simulink model "sampleModel349"  (R2021b)
settings: Solver=VariableStepAuto  StartTime=0.0  StopTime=10.0  RelTol=1e-3
undefined symbols (not defined in the file or in its folder): Newton, Raphson
libraries: simulink x12, slpidlib x2, simulink_need_slupdate x2
settings Model: Creator=user  LastModifiedBy=user

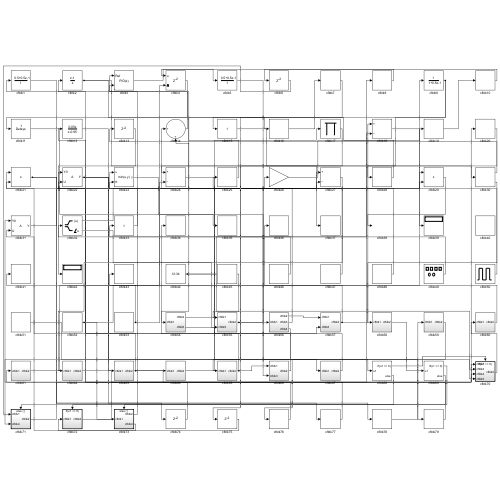
[thumbnail: Simulink's stored preview of the top-level diagram]
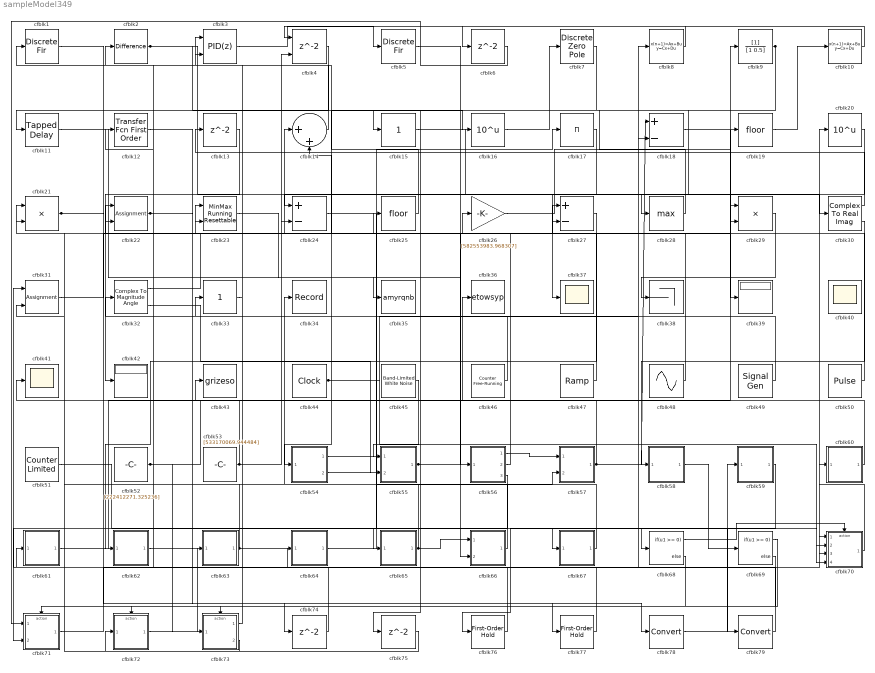
== system sampleModel349 ==
  cfblk1 : DiscreteFir  SampleTime=1
  cfblk10 : DiscreteStateSpace
  cfblk11 : simulink/Discrete/Tapped Delay  vinit=0.0  samptime=-1  NumDelays=1  DelayOrder=Oldest  includeCurrent=off
  cfblk12 : simulink/Discrete/Transfer Fcn First Order  PoleZ=0.95  ICPrevOutput=0.0  DoSatur=off
  cfblk{6,13,74..75} (4 alike) : Delay  SampleTime=1
  cfblk14 : Sum  Inputs=|++
  cfblk15 : simulink/Math Operations/Slider Gain  gain=1  low=0  high=2
  cfblk16 : Math  Operator=10^u  SaturateOnIntegerOverflow=on
  cfblk17 : Product  Inputs=*
  cfblk18 : Sum  Inputs=+-
  cfblk19 : Rounding
  cfblk2 : simulink/Discrete/Difference  ICPrevInput=0.0  OutMin=[]  OutMax=[]  OutDataTypeStr=Inherit: Inherit via back propagation  OutDataType=fixdt(1, 16)  OutScaling=2^-10  DoSatur=off
  cfblk20 : Math  Operator=10^u  SaturateOnIntegerOverflow=on
  cfblk21 : Product
  cfblk22 : Assignment  DiagnosticForDimensions=Warning  IndexOptions=Index vector (dialog)  Indices=1  OutputSizes=1
  cfblk23 : simulink/Math Operations/MinMax Running Resettable  Function=min  vinit=0.0
  cfblk24 : Sum  Inputs=+-
  cfblk25 : Rounding
  cfblk26 : Gain  Gain=[582553983.968307]
  cfblk27 : Sum  Inputs=+-
  cfblk28 : MinMax  Function=max
  cfblk29 : Product
  cfblk3 : slpidlib/PID Controller (2DOF)  Controller=PID  Form=Parallel  TimeDomain=Discrete-time  UseExternalTs=off  SampleTime=1  IntegratorMethod=Forward Euler  FilterMethod=Forward Euler  ControllerParametersSource=internal  P=1  I=1  D=0  UseFilter=on  N=100  b=1  c=1  TunerSelectOption=Transfer Function Based (PID Tuner App)  InitialConditionSource=internal  InitialConditionForIntegrator=0  InitialConditionForFilter=0  DifferentiatorICPrevScaledInput=0  ExternalReset=none  TrackingMode=off  Kt=1  LimitOutput=off  SatLimitsSource=internal  UpperSaturationLimit=inf  LowerSaturationLimit=-inf  LinearizeAsGain=off  AntiWindupMode=none  Kb=1  POutMin=[]  POutMax=[]  IOutMin=[]  IOutMax=[]  DOutMin=[]  DOutMax=[]  NOutMin=[]  NOutMax=[]  bOutMin=[]  bOutMax=[]  cOutMin=[]  cOutMax=[]  SumOutMin=[]  SumOutMax=[]  SaturationOutMin=[]  SaturationOutMax=[]  PParamMin=[]  PParamMax=[]  IParamMin=[]  IParamMax=[]  DParamMin=[]  DParamMax=[]  NParamMin=[]  NParamMax=[]  bParamMin=[]  bParamMax=[]  cParamMin=[]  cParamMax=[]  KbParamMin=[]  KbParamMax=[]  KtParamMin=[]  KtParamMax=[]  KbOutMin=[]  KbOutMax=[]  KtOutMin=[]  KtOutMax=[]  IntegratorOutMin=[]  IntegratorOutMax=[]  FilterOutMin=[]  FilterOutMax=[]  SumI1OutMin=[]  SumI1OutMax=[]  SumI2OutMin=[]  SumI2OutMax=[]  SumI3OutMin=[]  SumI3OutMax=[]  SumI4OutMin=[]  SumI4OutMax=[]  SumDOutMin=[]  SumDOutMax=[]  Sum1OutMin=[]  Sum1OutMax=[]  Sum2OutMin=[]  Sum2OutMax=[]  Sum3OutMin=[]  Sum3OutMax=[]  DifferentiatorOutMin=[]  DifferentiatorOutMax=[]  FilterDiffOutCoefMin=[]  FilterDiffOutCoefMax=[]  ReciprocalOutMin=[]  ReciprocalOutMax=[]  SumDenOutMin=[]  SumDenOutMax=[]  SumNumOutMin=[]  SumNumOutMax=[]  DivideOutMin=[]  DivideOutMax=[]  UdiffTsProdOutMin=[]  UdiffTsProdOutMax=[]  NTsProdOutMin=[]  NTsProdOutMax=[]  UintegralTsProdOutMin=[]  UintegralTsProdOutMax=[]  UngainTsProdOutMin=[]  UngainTsProdOutMax=[]  IntegratorContinuousStateAttributes=''  IntegratorStateMustResolveToSignalObject=off  IntegratorRTWStateStorageClass=Auto  FilterContinuousStateAttributes=''  FilterStateMustResolveToSignalObject=off  FilterRTWStateStorageClass=Auto  ParallelPVariant=InternalParameters  IdealPVariant=Disabled  IVariant=InternalParameters  DVariant=InternalParameters  bVariant=InternalParameters  cVariant=InternalParameters  IntegratorVariant=Discrete  SatVariant=Disabled  AWVariant=Passthrough  PCopyVariant=Disabled  TRVariant=Disabled  FdbkBlocksVariant=Forward  IdealPFdbkVariant=Disabled  SatFdbkVariant=Disabled  DerivativeFilterVariant=ForwardEulerFilter  NVariant=InternalParameters  NCopyVariant=Disabled  FilterICVariant=InternalICsFilter  IntegratorICVariant=InternalICs  ExternalResetVariant=Disabled  TRSumVariant=Passthrough  SumFdbkVariant=Disabled  SumVariant=Sum_PID  TsampFilterVariant=InternalTs  TsampNgainVariant=Passthrough  TsampIntegralVariant=Passthrough  ExternalSaturationOutDataTypeStr=Inherit: Same as second input
      settings: SourceProductBaseCode=SL
  cfblk30 : ComplexToRealImag
  cfblk31 : Assignment  DiagnosticForDimensions=Warning  IndexOptions=Index vector (dialog)  Indices=1  OutputSizes=1
  cfblk32 : ComplexToMagnitudeAngle
  cfblk33 : simulink/Math Operations/Slider Gain  gain=1  low=0  high=2
  cfblk34 : Record  FileSettingsInternal="{\"entries\":[{\"content\":{\"excelSettings\":{\"content\":{},\"type\":\"Streamout.ExcelSettings\"}},\"type\":\"Streamout.FileSettingStorage\",\"uuid\":\"f71aceab-5a60-49d6-a025-645f4f33ca44\"}],\"packageUris\":[\"http://schema.mathworks.com/mf0/streamout_blocks/R2020a\"],\"version\":\"1.0\"}"  SignalsInternal="{\"entries\":[{\"content\":{\"signals\":[{\"content\":{\"blockPath\":[\"sampleModel349/cfblk34\"],\"channel\":[],\"dimensions\":[1],\"domain\":\"sampleModel349/cfblk34\",\"lineColor\":\"#d95319\",\"plots\":[1],\"port\":1,\"sid\":[\"\"],\"signalID\":14601,\"signalName\":\"cfblk67\"},\"type\":\"RecordBlkView.Signal\",\"uuid\":\"4f28f7ec-e5ea-41ac-ba8a-1c5bf7ad2562\"}]},\"type\":\"RecordBlkView.InputSignals\",\"uuid\":\"3db0044d-db04-4044-a744-d9451d8b6dbf\"}],\"packageUris\":[\"http://schema.mathworks.com/mf0/streamout_blocks/R2020a\"],\"version\":\"1.0\"}"  VisualizationBindings="{\"sparklinesplugin\":{\"info\":[{\"bindingParametersList\":[],\"subplotID\":1}]}}"
  cfblk35 : ToWorkspace  VariableName=amyrqnb  SaveFormat=Timeseries  SampleTime=-1
  cfblk36 : ToWorkspace  VariableName=etowsyp  SaveFormat=Timeseries  SampleTime=-1
  cfblk37 : Scope
  cfblk38 : Terminator
  cfblk39 : Display
  cfblk4 : Delay  ShowEnablePort=on  SampleTime=1
      settings: InputPortMap=u0,e6
  cfblk40 : Scope
      settings: Floating=on
  cfblk41 : Scope
  cfblk42 : Display
  cfblk43 : ToWorkspace  VariableName=grizeso  SaveFormat=Timeseries  SampleTime=-1
  cfblk44 : DigitalClock
  cfblk45 : simulink/Sources/Band-Limited White Noise  Cov=[8754681935.924770]  Ts=0.1  seed=[7344934764.000000]
  cfblk46 : simulink/Sources/Counter Free-Running  NumBits=[11.000000]  tsamp=-1
  cfblk47 : simulink/Sources/Ramp  slope=[7962.295624]  start=[45.118669]  InitialOutput=[46132.244628]
  cfblk48 : Sin  Amplitude=[-585222827.413026]  Bias=[408906363.797786]  SampleTime=0
  cfblk49 : SignalGenerator  Amplitude=[-354647075.884674]
  cfblk5 : DiscreteFir  SampleTime=1
  cfblk50 : DiscretePulseGenerator  PulseType=Time based  Amplitude=[-738225747.872744]  Period=[73691068.508407]  PulseWidth=5  PhaseDelay=[9.000000]
  cfblk51 : simulink/Sources/Counter Limited  uplimit=[482.000000]  tsamp=-1
  cfblk52 : Constant  Value=[222412271.325236]  SampleTime=1
  cfblk53 : Constant  Value=[533170069.944484]  SampleTime=1
  cfblk54 : Subsystem
  cfblk55 : Subsystem
  cfblk56 : Subsystem
  cfblk57 : Subsystem
  cfblk58 : Subsystem
  cfblk59 : Subsystem
  cfblk60 : Subsystem
  cfblk61 : Subsystem
  cfblk62 : Subsystem
  cfblk63 : Subsystem
  cfblk64 : Subsystem
  cfblk65 : Subsystem
  cfblk66 : Subsystem
  cfblk67 : Subsystem
  cfblk68 : If  IfExpression=u1 >= 0  SampleTime=1
  cfblk69 : If  IfExpression=u1 >= 0  SampleTime=1
  cfblk7 : DiscreteZeroPole  Poles=[0 0.5]  Gain=1
  cfblk70 : Subsystem  TreatAsAtomicUnit=on
  cfblk71 : Subsystem  TreatAsAtomicUnit=on
  cfblk72 : Subsystem  TreatAsAtomicUnit=on
  cfblk73 : Subsystem  TreatAsAtomicUnit=on
  cfblk76 : simulink_need_slupdate/First-Order Hold  DisableCoverage=on  Ts=1
      settings: SourceProductBaseCode=SL
  cfblk77 : simulink_need_slupdate/First-Order Hold  DisableCoverage=on  Ts=1
      settings: SourceProductBaseCode=SL
  cfblk78 : DataTypeConversion
  cfblk79 : DataTypeConversion
  cfblk8 : DiscreteStateSpace
  cfblk9 : DiscreteFilter  SampleTime=1
  wires:
  cfblk25/1 -> cfblk3/1
  cfblk24/1 -> cfblk68/1
  cfblk46/1 -> cfblk33/1
  cfblk64/1(cfblk2) -> cfblk17/1
  cfblk62/1(cfblk2) -> cfblk20/1
  cfblk55/1(cfblk2) -> cfblk56/1(cfblk1), cfblk27/1
  cfblk10/1 -> cfblk6/1
  cfblk3/1 -> cfblk5/1
  cfblk28/1 -> cfblk15/1
  cfblk13/1 -> cfblk42/1
  cfblk6/1 -> cfblk71/1(cfblk1)
  cfblk5/1 -> cfblk67/1(cfblk1)
  cfblk47/1 -> cfblk14/1
  cfblk54/1(cfblk2) -> cfblk26/1
  cfblk67/1(cfblk2) -> cfblk34/1
  cfblk48/1 -> cfblk25/1
  cfblk7/1 -> cfblk24/1
  cfblk15/1 -> cfblk37/1
  cfblk23/1 -> cfblk35/1
  cfblk49/1 -> cfblk32/1
  cfblk73/1(cfblk2) -> cfblk23/1
  cfblk61/1(cfblk2) -> cfblk9/1
  cfblk57/1(cfblk2) -> cfblk18/1, cfblk36/1
  cfblk2/1 -> cfblk30/1, cfblk16/1
  cfblk4/1 -> cfblk11/1
  cfblk19/1 -> cfblk10/1
  cfblk30/1 -> cfblk13/1
  cfblk65/1(cfblk2) -> cfblk66/1(cfblk1), cfblk22/2
  cfblk27/1 -> cfblk62/1(cfblk1)
  cfblk56/1(cfblk2) -> cfblk57/1(cfblk1)
  cfblk58/1(cfblk2) -> cfblk69/1
  cfblk11/1 -> cfblk66/2(cfblk3)
  cfblk56/2(cfblk3) -> cfblk21/1
  cfblk14/1 -> cfblk1/1
  cfblk50/1 -> cfblk14/2
  cfblk52/1 -> cfblk24/2, cfblk73/1(cfblk1)
  cfblk33/1 -> cfblk3/2
  cfblk73/2(cfblk4) -> cfblk61/1(cfblk1)
  cfblk22/1 -> cfblk63/1(cfblk1), cfblk27/2, cfblk70/4(cfblk5)
  cfblk72/1(cfblk2) -> cfblk18/2
  cfblk8/1 -> cfblk4/1
  cfblk21/1 -> cfblk23/2, cfblk74/1
  cfblk20/1 -> cfblk54/1(cfblk1)
  cfblk63/1(cfblk2) -> cfblk21/2, cfblk70/3(cfblk4), cfblk64/1(cfblk1)
  cfblk56/3(cfblk4) -> cfblk71/2(cfblk4)
  cfblk45/1 -> cfblk55/1(cfblk1)
  cfblk60/1(cfblk2) -> cfblk43/1
  cfblk18/1 -> cfblk39/1
  cfblk70/1(cfblk2) -> cfblk60/1(cfblk1)
  cfblk16/1 -> cfblk7/1
  cfblk31/1 -> cfblk29/1
  cfblk32/1 -> cfblk29/2
  cfblk9/1 -> cfblk65/1(cfblk1), cfblk28/1
  cfblk29/1 -> cfblk38/1
  cfblk66/1(cfblk2) -> cfblk22/1
  cfblk71/1(cfblk2) -> cfblk70/1(cfblk1)
  cfblk54/2(cfblk5) -> cfblk57/2(cfblk3)
  cfblk26/1 -> cfblk19/1
  cfblk53/1 -> cfblk4/2, cfblk41/1
  cfblk44/1 -> cfblk8/1, cfblk70/2(cfblk3)
  cfblk30/2 -> cfblk58/1(cfblk1)
  cfblk32/2 -> cfblk55/2(cfblk5)
  cfblk68/1 -> cfblk70/Action
  cfblk68/2 -> cfblk71/Action
  cfblk69/1 -> cfblk72/Action
  cfblk69/2 -> cfblk73/Action
  cfblk74/1 -> cfblk2/1
  cfblk17/1 -> cfblk75/1
  cfblk75/1 -> cfblk72/1(cfblk1)
  cfblk59/1(cfblk2) -> cfblk76/1
  cfblk76/1 -> cfblk31/1
  cfblk1/1 -> cfblk77/1
  cfblk77/1 -> cfblk31/2
  cfblk12/1 -> cfblk78/1
  cfblk78/1 -> cfblk59/1(cfblk1)
  cfblk51/1 -> cfblk79/1
  cfblk79/1 -> cfblk12/1

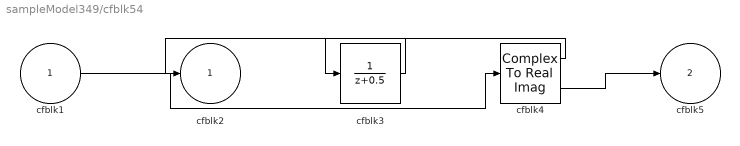
== system sampleModel349/cfblk54 ==
  cfblk1 : Inport
  cfblk3 : DiscreteTransferFcn  SampleTime=1
  cfblk4 : ComplexToRealImag
  cfblk2 : Outport
  cfblk5 : Outport  Port=2
  wires:
  cfblk4/1 -> cfblk3/1
  cfblk1/1 -> cfblk4/1
  cfblk3/1 -> cfblk2/1
  cfblk4/2 -> cfblk5/1

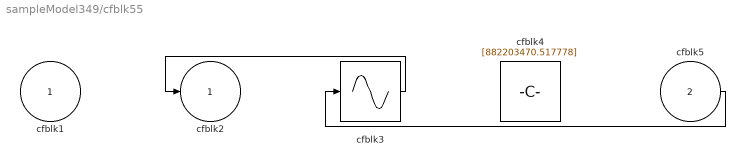
== system sampleModel349/cfblk55 ==
  cfblk1 : Inport
  cfblk5 : Inport  Port=2
  cfblk3 : Sin  TimeSource=Use external signal  SampleTime=0
  cfblk4 : Constant  Value=[882203470.517778]  SampleTime=1
  cfblk2 : Outport
  wires:
  cfblk3/1 -> cfblk2/1
  cfblk5/1 -> cfblk3/1

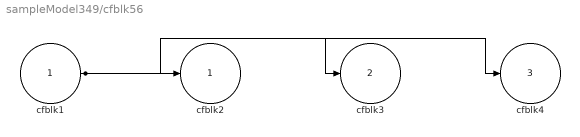
== system sampleModel349/cfblk56 ==
  cfblk1 : Inport
  cfblk2 : Outport
  cfblk3 : Outport  Port=2
  cfblk4 : Outport  Port=3
  wires:
  cfblk1/1 -> cfblk2/1, cfblk3/1, cfblk4/1

== system sampleModel349/cfblk57 ==
  cfblk1 : Inport
  cfblk3 : Inport  Port=2
  cfblk2 : Outport
  wires:
  cfblk1/1 -> cfblk2/1

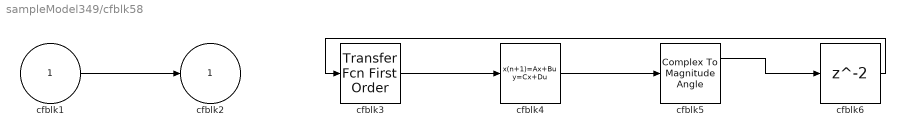
== system sampleModel349/cfblk58 ==
  cfblk1 : Inport
  cfblk3 : simulink/Discrete/Transfer Fcn First Order  PoleZ=0.95  ICPrevOutput=0.0  DoSatur=off
  cfblk4 : DiscreteStateSpace
  cfblk5 : ComplexToMagnitudeAngle
  cfblk6 : Delay  SampleTime=1
  cfblk2 : Outport
  wires:
  cfblk1/1 -> cfblk2/1
  cfblk3/1 -> cfblk4/1
  cfblk4/1 -> cfblk5/1
  cfblk5/1 -> cfblk6/1
  cfblk6/1 -> cfblk3/1

== system sampleModel349/cfblk59 ==
  cfblk1 : Inport
  cfblk3 : Sqrt  Operator=rSqrt  AlgorithmType=Newton-Raphson  SaturateOnIntegerOverflow=on
  cfblk2 : Outport
  wires:
  cfblk1/1 -> cfblk3/1
  cfblk3/1 -> cfblk2/1

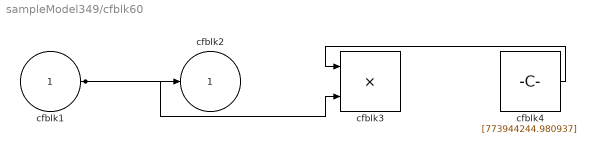
== system sampleModel349/cfblk60 ==
  cfblk1 : Inport
  cfblk3 : Product  Inputs=**
  cfblk4 : Constant  Value=[773944244.980937]  SampleTime=1
  cfblk2 : Outport
  wires:
  cfblk4/1 -> cfblk3/1
  cfblk1/1 -> cfblk2/1, cfblk3/2

== system sampleModel349/cfblk61 ==
  cfblk1 : Inport
  cfblk3 : UnitDelay  HasFrameUpgradeWarning=on
  cfblk2 : Outport
  wires:
  cfblk1/1 -> cfblk2/1, cfblk3/1

== system sampleModel349/cfblk62 ==
  cfblk1 : Inport
  cfblk3 : DiscreteFir  SampleTime=1
  cfblk4 : ComplexToRealImag
  cfblk2 : Outport
  wires:
  cfblk3/1 -> cfblk2/1
  cfblk1/1 -> cfblk3/1, cfblk4/1

== system sampleModel349/cfblk63 ==
  cfblk1 : Inport
  cfblk3 : Sum  Inputs=+-
  cfblk2 : Outport
  wires:
  cfblk1/1 -> cfblk2/1, cfblk3/1, cfblk3/2

== system sampleModel349/cfblk64 ==
  cfblk1 : Inport
  cfblk3 : Signum
  cfblk4 : ComplexToRealImag
  cfblk2 : Outport
  wires:
  cfblk4/1 -> cfblk3/1
  cfblk3/1 -> cfblk2/1
  cfblk1/1 -> cfblk4/1

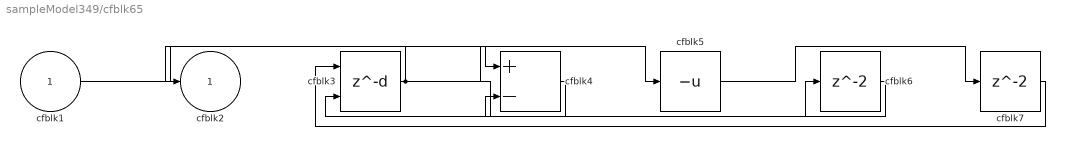
== system sampleModel349/cfblk65 ==
  cfblk1 : Inport
  cfblk3 : Delay  DelayLengthSource=Input port  SampleTime=1
      settings: InputPortMap=u0,p1
  cfblk4 : Sum  Inputs=+-
  cfblk5 : UnaryMinus
  cfblk6 : Delay  SampleTime=1
  cfblk7 : Delay  SampleTime=1
  cfblk2 : Outport
  wires:
  cfblk4/1 -> cfblk3/2
  cfblk1/1 -> cfblk4/1
  cfblk3/1 -> cfblk2/1, cfblk5/1, cfblk6/1
  cfblk6/1 -> cfblk4/2
  cfblk5/1 -> cfblk7/1
  cfblk7/1 -> cfblk3/1

== system sampleModel349/cfblk66 ==
  cfblk1 : Inport
  cfblk3 : Inport  Port=2
  cfblk2 : Outport
  wires:
  cfblk3/1 -> cfblk2/1

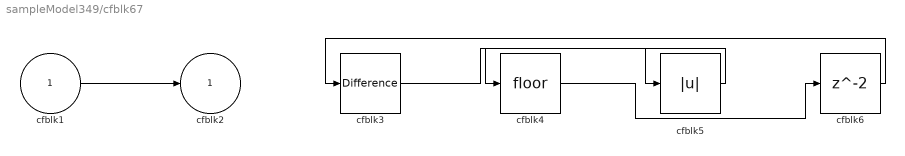
== system sampleModel349/cfblk67 ==
  cfblk1 : Inport
  cfblk3 : simulink/Discrete/Difference  ICPrevInput=0.0  OutMin=[]  OutMax=[]  OutDataTypeStr=Inherit: Inherit via back propagation  OutDataType=fixdt(1, 16)  OutScaling=2^-10  DoSatur=off
  cfblk4 : Rounding
  cfblk5 : Abs
  cfblk6 : Delay  SampleTime=1
  cfblk2 : Outport
  wires:
  cfblk5/1 -> cfblk4/1
  cfblk3/1 -> cfblk5/1
  cfblk1/1 -> cfblk2/1
  cfblk4/1 -> cfblk6/1
  cfblk6/1 -> cfblk3/1

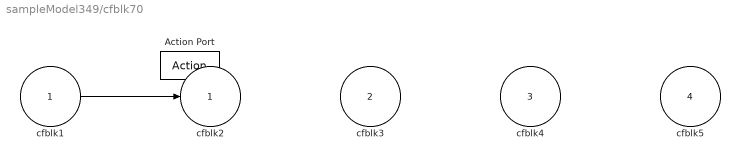
== system sampleModel349/cfblk70 ==
  cfblk1 : Inport
  cfblk3 : Inport  Port=2
  cfblk4 : Inport  Port=3
  cfblk5 : Inport  Port=4
  Action Port : ActionPort  ActionPortLabel=if(u1 >= 0)
  cfblk2 : Outport
  wires:
  cfblk1/1 -> cfblk2/1

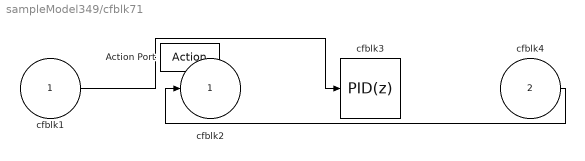
== system sampleModel349/cfblk71 ==
  cfblk1 : Inport
  cfblk4 : Inport  Port=2
  Action Port : ActionPort  ActionPortLabel=else
  cfblk3 : slpidlib/PID Controller  Controller=PID  Form=Parallel  TimeDomain=Discrete-time  UseExternalTs=off  SampleTime=-1  IntegratorMethod=Forward Euler  FilterMethod=Forward Euler  ControllerParametersSource=internal  P=1  I=1  D=0  UseFilter=on  N=100  TunerSelectOption=Transfer Function Based (PID Tuner App)  InitialConditionSource=internal  InitialConditionForIntegrator=0  InitialConditionForFilter=0  DifferentiatorICPrevScaledInput=0  ExternalReset=none  TrackingMode=off  Kt=1  LimitOutput=off  SatLimitsSource=internal  UpperSaturationLimit=inf  LowerSaturationLimit=-inf  LinearizeAsGain=off  AntiWindupMode=none  Kb=1  POutMin=[]  POutMax=[]  IOutMin=[]  IOutMax=[]  DOutMin=[]  DOutMax=[]  NOutMin=[]  NOutMax=[]  SumOutMin=[]  SumOutMax=[]  SaturationOutMin=[]  SaturationOutMax=[]  PParamMin=[]  PParamMax=[]  IParamMin=[]  IParamMax=[]  DParamMin=[]  DParamMax=[]  NParamMin=[]  NParamMax=[]  KbParamMin=[]  KbParamMax=[]  KtParamMin=[]  KtParamMax=[]  KbOutMin=[]  KbOutMax=[]  KtOutMin=[]  KtOutMax=[]  IntegratorOutMin=[]  IntegratorOutMax=[]  FilterOutMin=[]  FilterOutMax=[]  SumI1OutMin=[]  SumI1OutMax=[]  SumI2OutMin=[]  SumI2OutMax=[]  SumI3OutMin=[]  SumI3OutMax=[]  SumI4OutMin=[]  SumI4OutMax=[]  SumDOutMin=[]  SumDOutMax=[]  DifferentiatorOutMin=[]  DifferentiatorOutMax=[]  FilterDiffOutCoefMin=[]  FilterDiffOutCoefMax=[]  ReciprocalOutMin=[]  ReciprocalOutMax=[]  SumDenOutMin=[]  SumDenOutMax=[]  SumNumOutMin=[]  SumNumOutMax=[]  DivideOutMin=[]  DivideOutMax=[]  UdiffTsProdOutMin=[]  UdiffTsProdOutMax=[]  NTsProdOutMin=[]  NTsProdOutMax=[]  UintegralTsProdOutMin=[]  UintegralTsProdOutMax=[]  UngainTsProdOutMin=[]  UngainTsProdOutMax=[]  IntegratorContinuousStateAttributes=''  IntegratorStateMustResolveToSignalObject=off  IntegratorRTWStateStorageClass=Auto  FilterContinuousStateAttributes=''  FilterStateMustResolveToSignalObject=off  FilterRTWStateStorageClass=Auto  ParallelPVariant=InternalParameters  IdealPVariant=Disabled  IVariant=InternalParameters  DVariant=InternalParameters  IntegratorVariant=Discrete  SatVariant=Disabled  AWVariant=Passthrough  PCopyVariant=Disabled  TRVariant=Disabled  FdbkBlocksVariant=Forward  IdealPFdbkVariant=Disabled  SatFdbkVariant=Disabled  DerivativeFilterVariant=ForwardEulerFilter  NVariant=InternalParameters  NCopyVariant=Disabled  FilterICVariant=InternalICsFilter  IntegratorICVariant=InternalICs  ExternalResetVariant=Disabled  TRSumVariant=Passthrough  SumFdbkVariant=Disabled  SumVariant=Sum_PID  TsampFilterVariant=InternalTs  TsampNgainVariant=Passthrough  TsampIntegralVariant=Passthrough  ExternalSaturationOutDataTypeStr=Inherit: Same as second input
  cfblk2 : Outport
  wires:
  cfblk4/1 -> cfblk2/1
  cfblk1/1 -> cfblk3/1

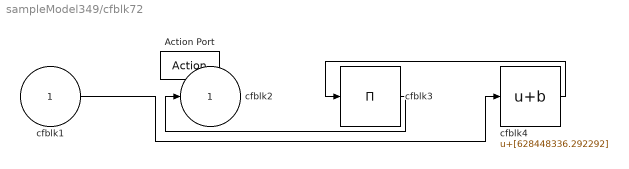
== system sampleModel349/cfblk72 ==
  cfblk1 : Inport
  Action Port : ActionPort  ActionPortLabel=if(u1 >= 0)
  cfblk3 : Product  Inputs=*
  cfblk4 : Bias  Bias=[628448336.292292]
  cfblk2 : Outport
  wires:
  cfblk3/1 -> cfblk2/1
  cfblk4/1 -> cfblk3/1
  cfblk1/1 -> cfblk4/1

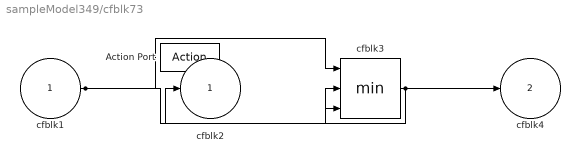
== system sampleModel349/cfblk73 ==
  cfblk1 : Inport
  Action Port : ActionPort  ActionPortLabel=else
  cfblk3 : MinMax  Inputs=3
  cfblk2 : Outport
  cfblk4 : Outport  Port=2
  wires:
  cfblk1/1 -> cfblk3/1, cfblk3/2, cfblk3/3
  cfblk3/1 -> cfblk4/1, cfblk2/1
